simulink model "Ctrl_For_HRV_20260625"  (R2024b)
settings: Solver=ode4  StartTime=0.0  StopTime=22  FixedStep=0.02  RelTol=1e-3
InitFcn:
  | Parameter;
undefined symbols (not defined in the file or in its folder): CCI_DUI_AngleRate_Controller, CCI_DUI_FlowAngle_Controller, fhan, h_alpha, h_beta, h_miu, h_p, h_q, h_r, PNG_2026_6_23, r_alpha, r_beta, r_miu, r_p, r_q, r_r, xishu, xishu_D_0, xishu_L_0, xishu_l_0, xishu_m_0, xishu_n_0, xishu_Y_0
libraries: simulink x60
(part 3 of 8)

== system Ctrl_For_HRV_20260625/Vehicle_4/AngleRate_ESO_v4 ==
  Add{,1..5} (6 alike) : Sum  Inputs=+-
  Demux : Demux  Outputs=6
  Mux{,1..5} (6 alike) : Mux  Inputs=2
  Mux10 : Mux  Inputs=6
  S-Function : S-Function  FunctionName=fastloop_ESO  SFunctionDeploymentMode=off  EnableBusSupport=off
  Scope_p_hat : Scope
  Scope_p_hat_error : Scope
  Scope_phi_p_hat : Scope
  Scope_phi_p_hat_error : Scope
  Scope_phi_q_hat : Scope
  Scope_phi_q_hat_error : Scope
  Scope_phi_r_hat : Scope
  Scope_phi_r_hat_error : Scope
  Scope_q_hat : Scope
  Scope_q_hat_error : Scope
  Scope_r_hat : Scope
  Scope_r_hat_error : Scope
  tag scope: p_hat_v4=global, phi_p_hat_v4=global, phi_q_hat_v4=global, phi_r_hat_v4=global, q_hat_v4=global, r_hat_v4=global
  wires:
  Add5/1 -> Scope_phi_r_hat_error/1
  [phi_r_hat_v4] -> Add5/2
  [phi_r_v4] -> Add5/1
  Add4/1 -> Scope_phi_q_hat_error/1
  [phi_q_hat_v4] -> Add4/2
  [phi_q_v4] -> Add4/1
  Add3/1 -> Scope_phi_p_hat_error/1
  [phi_p_hat_v4] -> Add3/2
  [phi_p_v4] -> Add3/1
  Add2/1 -> Scope_r_hat_error/1
  [r_hat_v4] -> Add2/2
  [r_noise_v4] -> Add2/1
  Add1/1 -> Scope_q_hat_error/1
  [q_hat_v4] -> Add1/2
  [q_noise_v4] -> Add1/1
  Add/1 -> Scope_p_hat_error/1
  [p_hat_v4] -> Add/2
  [p_noise_v4] -> Add/1
  Mux3/1 -> Scope_phi_p_hat/1
  [phi_p_v4] -> Mux3/1
  [phi_p_hat_v4] -> Mux3/2
  [phi_q_v4] -> Mux4/1
  [phi_q_hat_v4] -> Mux4/2
  Mux4/1 -> Scope_phi_q_hat/1
  [phi_r_v4] -> Mux5/1
  [phi_r_hat_v4] -> Mux5/2
  Mux5/1 -> Scope_phi_r_hat/1
  Mux2/1 -> Scope_r_hat/1
  [r_hat_v4] -> Mux2/2
  [r_noise_v4] -> Mux2/1
  Mux1/1 -> Scope_q_hat/1
  [q_hat_v4] -> Mux1/2
  [q_noise_v4] -> Mux1/1
  [p_hat_v4] -> Mux/2
  [p_noise_v4] -> Mux/1
  Mux/1 -> Scope_p_hat/1
  [b_r_v4] -> Mux10/6
  [p_noise_v4] -> Mux10/1
  Demux/6 -> [phi_r_hat_v4]
  Mux10/1 -> S-Function/1
  Demux/4 -> [phi_p_hat_v4]
  Demux/3 -> [r_hat_v4]
  Demux/1 -> [p_hat_v4]
  Demux/5 -> [phi_q_hat_v4]
  S-Function/1 -> Demux/1
  [b_p_v4] -> Mux10/4
  Demux/2 -> [q_hat_v4]
  [q_noise_v4] -> Mux10/2
  [r_noise_v4] -> Mux10/3
  [b_q_v4] -> Mux10/5

== system Ctrl_For_HRV_20260625/Vehicle_4/Error_Model ==
  Delay : Delay  DelayLength=1
  Delay1 : Delay  DelayLength=1
  Delay2 : Delay  DelayLength=1
  Demux : Demux  Outputs=9
  Mux : Mux  Inputs=33
  S-Function : S-Function  FunctionName=Error_Model  SFunctionDeploymentMode=off  EnableBusSupport=off
  TD_alpha1 : Subsystem
  TD_alpha2 : Subsystem
  TD_alpha3 : Subsystem
  tag scope: dot_e_wd_1=global, dot_e_wd_2=global, dot_e_wd_3=global, e_alpha=global, e_beta=global, e_miu=global, e_w_1=global, e_w_2=global, e_w_3=global, e_wd_1=global, e_wd_2=global, e_wd_3=global
  wires:
  [theta] -> Mux/33
  [r] -> Mux/32
  [q] -> Mux/31
  [p] -> Mux/30
  [miu] -> Mux/29
  [beta] -> Mux/28
  [alpha] -> Mux/27
  [delta_r] -> Mux/3
  [delta_e] -> Mux/2
  [delta_a] -> Mux/1
  [dot_e_wd_3] -> Mux/26
  [dot_e_wd_2] -> Mux/25
  [dot_e_wd_1] -> Mux/24
  TD_alpha3/1(dot_e_wd_3) -> [dot_e_wd_3]
  [e_wd_3] -> TD_alpha3/1(e_wd_3)
  [e_wd_2] -> TD_alpha2/1(e_wd_2)
  TD_alpha2/1(dot_e_wd_2) -> [dot_e_wd_2]
  TD_alpha1/1(dot_e_wd_1) -> [dot_e_wd_1]
  [e_wd_1] -> TD_alpha1/1(e_wd_1)
  Delay2/1 -> Mux/23
  [e_wd_3] -> Delay2/1
  [e_wd_2] -> Delay1/1
  Delay1/1 -> Mux/22
  Delay/1 -> Mux/21
  [e_wd_1] -> Delay/1
  Demux/7 -> [e_wd_1]
  Demux/8 -> [e_wd_2]
  Demux/9 -> [e_wd_3]
  Demux/6 -> [e_w_3]
  Demux/5 -> [e_w_2]
  Demux/4 -> [e_w_1]
  Demux/3 -> [e_miu]
  Demux/2 -> [e_beta]
  Demux/1 -> [e_alpha]
  S-Function/1 -> Demux/1
  [ddot_miu_c] -> Mux/20
  [ddot_beta_c] -> Mux/19
  [ddot_alpha_c] -> Mux/18
  [dot_alpha_c] -> Mux/15
  [dot_beta_c] -> Mux/16
  [dot_miu_c] -> Mux/17
  [miu_c] -> Mux/14
  [beta_c] -> Mux/13
  [alpha_c] -> Mux/12
  [V] -> Mux/11
  [H] -> Mux/10
  [C_m_d] -> Mux/8
  [C_n_d] -> Mux/9
  [C_Y_d] -> Mux/6
  [C_L_d] -> Mux/4
  [C_D_d] -> Mux/5
  [C_l_d] -> Mux/7
  Mux/1 -> S-Function/1

== system Ctrl_For_HRV_20260625/Vehicle_4/FlowAngle_Controller_v4 ==
  alpha_d : Inport
  beta_d : Inport  Port=2
  miu_d : Inport  Port=3
  Demux : Demux  Outputs=9
  From12 : From  Commented=on  GotoTag=dot_alpha_c  TagVisibility=global
  From13 : From  Commented=on  GotoTag=dot_beta_c  TagVisibility=global
  From14 : From  Commented=on  GotoTag=dot_miu_c  TagVisibility=global
  Goto6 : Goto  Commented=on  GotoTag=ddot_alpha_c  TagVisibility=global
  Goto7 : Goto  Commented=on  GotoTag=ddot_beta_c  TagVisibility=global
  Goto8 : Goto  Commented=on  GotoTag=ddot_miu_c  TagVisibility=global
  Interpreted MATLAB Function : MATLABFcn  MATLABFcn=CCI_DUI_FlowAngle_Controller(u(1),u(2),u(3),u(4),u(5),u(6),u(7),u(8),u(9),u(10),u(11),u(12),u(13),u(14),u(15),u(16),u(17),u(18))  OutputDimensions=9
  Mux : Mux  Inputs=18
  Mux1 : Mux  Inputs=3
  Mux2 : Mux  Inputs=3
  Scope_CCI_FlowAngle : Scope
  Scope_DUI_FlowAngle : Scope
  Scope_alpha_d : Scope
  Scope_beta_d : Scope
  Scope_miu_d : Scope
  TD_alpha : Subsystem
  TD_alpha2 : Subsystem
  TD_alpha3 : Subsystem  Commented=on
  TD_alpha4 : Subsystem  Commented=on
  TD_beta : Subsystem
  TD_beta1 : Subsystem
  TD_beta2 : Subsystem
  TD_dotalpha1 : Subsystem  Commented=on
  TD_miu : Subsystem
  p_d : Outport
  q_d : Outport  Port=2
  r_d : Outport  Port=3
  tag scope: alpha_c_v4=global, beta_c_v4=global, dot_alpha_c_v4=global, dot_beta_c_v4=global, dot_miu_c_v4=global, miu_c_v4=global
  wires:
  Demux/7 -> Mux2/1
  Demux/9 -> Mux2/3
  Demux/8 -> Mux2/2
  Mux2/1 -> Scope_DUI_FlowAngle/1
  Mux1/1 -> Scope_CCI_FlowAngle/1
  Demux/6 -> Mux1/3
  Demux/5 -> Mux1/2
  Demux/4 -> Mux1/1
  TD_alpha/1(alpha_c) -> Mux/13, [alpha_c_v4]
  TD_alpha4/1(ddot_miu_c) -> Goto8/1
  From14/1 -> TD_alpha4/1(dot_miu_c)
  TD_alpha3/1(ddot_beta_c) -> Goto7/1
  From13/1 -> TD_alpha3/1(dot_beta_c)
  TD_dotalpha1/1(ddot_alpha_c) -> Goto6/1
  From12/1 -> TD_dotalpha1/1(dot_alpha_c)
  [phi_miu_hat_v4] -> Mux/12
  [phi_beta_hat_v4] -> Mux/11
  [phi_alpha_hat_v4] -> Mux/10
  TD_miu/2(miu_c_dot) -> Mux/18, [dot_miu_c_v4]
  TD_miu/1(miu_c) -> Mux/17, [miu_c_v4]
  miu_d/1 -> TD_miu/1(miu_d), Scope_miu_d/1
  TD_beta/2(beta_c_dot) -> Mux/16, [dot_beta_c_v4]
  TD_beta/1(beta_c) -> Mux/15, [beta_c_v4]
  beta_d/1 -> TD_beta/1(beta_d), Scope_beta_d/1
  TD_alpha/2(alpha_c_dot) -> [dot_alpha_c_v4], Mux/14
  alpha_d/1 -> TD_alpha/1(alpha_d), Scope_alpha_d/1
  Demux/3 -> r_d/1
  Demux/2 -> q_d/1
  Demux/1 -> p_d/1
  Interpreted MATLAB Function/1 -> Demux/1
  Mux/1 -> Interpreted MATLAB Function/1
  [theta_v4] -> Mux/9
  [delta_a_v4] -> Mux/6
  [delta_e_v4] -> Mux/7
  [delta_r_v4] -> Mux/8
  [miu_noise_v4] -> Mux/5
  [beta_noise_v4] -> Mux/4
  [alpha_noise_v4] -> Mux/3
  [V_v4] -> Mux/2
  [H_v4] -> Mux/1

== system Ctrl_For_HRV_20260625/Vehicle_4/FlowAngle_ESO_v4 ==
  Add{,1..5} (6 alike) : Sum  Inputs=+-
  Demux : Demux  Outputs=6
  Mux{,1..5} (6 alike) : Mux  Inputs=2
  Mux10 : Mux  Inputs=6
  S-Function : S-Function  FunctionName=slowloop_ESO  SFunctionDeploymentMode=off  EnableBusSupport=off
  Scope_alpha_hat : Scope
  Scope_alpha_hat_error : Scope
  Scope_beta_hat : Scope
  Scope_beta_hat_error : Scope
  Scope_miu_hat : Scope
  Scope_miu_hat_error : Scope
  Scope_phi_alpha_hat : Scope
  Scope_phi_alpha_hat_error : Scope
  Scope_phi_beta_hat : Scope
  Scope_phi_beta_hat_error : Scope
  Scope_phi_miu_hat : Scope
  Scope_phi_miu_hat_error : Scope
  tag scope: alpha_hat_v4=global, beta_hat_v4=global, miu_hat_v4=global, phi_alpha_hat_v4=global, phi_beta_hat_v4=global, phi_miu_hat_v4=global
  wires:
  [phi_miu_hat_v4] -> Add5/2
  [phi_miu_v4] -> Add5/1
  Add5/1 -> Scope_phi_miu_hat_error/1
  Add4/1 -> Scope_phi_beta_hat_error/1
  [phi_beta_hat_v4] -> Add4/2
  [phi_beta_v4] -> Add4/1
  Add3/1 -> Scope_phi_alpha_hat_error/1
  [phi_alpha_hat_v4] -> Add3/2
  [phi_alpha_v4] -> Add3/1
  Add2/1 -> Scope_miu_hat_error/1
  [miu_hat_v4] -> Add2/2
  [miu_noise_v4] -> Add2/1
  Add1/1 -> Scope_beta_hat_error/1
  [beta_hat_v4] -> Add1/2
  [beta_noise_v4] -> Add1/1
  Add/1 -> Scope_alpha_hat_error/1
  [alpha_hat_v4] -> Add/2
  [alpha_noise_v4] -> Add/1
  Mux3/1 -> Scope_phi_alpha_hat/1
  [phi_alpha_v4] -> Mux3/1
  [phi_alpha_hat_v4] -> Mux3/2
  [phi_beta_v4] -> Mux4/1
  [phi_beta_hat_v4] -> Mux4/2
  Mux4/1 -> Scope_phi_beta_hat/1
  [phi_miu_v4] -> Mux5/1
  [phi_miu_hat_v4] -> Mux5/2
  Mux5/1 -> Scope_phi_miu_hat/1
  Mux2/1 -> Scope_miu_hat/1
  [miu_hat_v4] -> Mux2/2
  [miu_noise_v4] -> Mux2/1
  Mux1/1 -> Scope_beta_hat/1
  [beta_hat_v4] -> Mux1/2
  [beta_noise_v4] -> Mux1/1
  [alpha_hat_v4] -> Mux/2
  [alpha_noise_v4] -> Mux/1
  Mux/1 -> Scope_alpha_hat/1
  [b_miu_v4] -> Mux10/6
  [alpha_noise_v4] -> Mux10/1
  Demux/6 -> [phi_miu_hat_v4]
  Mux10/1 -> S-Function/1
  Demux/4 -> [phi_alpha_hat_v4]
  Demux/3 -> [miu_hat_v4]
  Demux/1 -> [alpha_hat_v4]
  Demux/5 -> [phi_beta_hat_v4]
  S-Function/1 -> Demux/1
  [b_alpha_v4] -> Mux10/4
  Demux/2 -> [beta_hat_v4]
  [beta_noise_v4] -> Mux10/2
  [miu_noise_v4] -> Mux10/3
  [b_beta_v4] -> Mux10/5

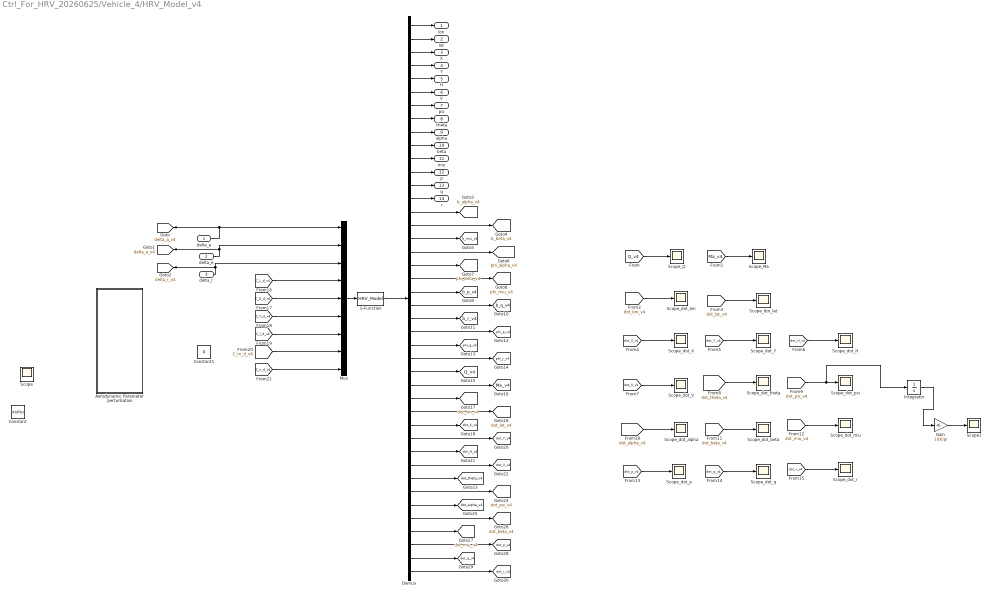
== system Ctrl_For_HRV_20260625/Vehicle_4/HRV_Model_v4 ==
  delta_a : Inport
  delta_e : Inport  Port=2
  delta_r : Inport  Port=3
  Aerodynamic Parameter perturbation : Subsystem
  Constant : Constant  Value=xishu  SampleTime=-1
  Constant1 : Constant  Value=0
  Demux : Demux  Outputs=14 + 12 + 2 + 14
  Gain : Gain  Gain=180/pi
  Integrator : Integrator  InitialCondition=[0 0 450 350 0 0 0.0349065850398866 0 0 0 0 0 0 0 0 0 0 0 0 0 0 0 0 0 0 0 0 0 0 0 0 0 0 0 0 0 0 0 0 0 0 0]
  Mux : Mux  Inputs=9
  S-Function : S-Function  FunctionName=HRV_Model  SFunctionDeploymentMode=off  EnableBusSupport=off
  Scope : Scope
  Scope1 : Scope
  Scope_Ma : Scope
  Scope_Q : Scope
  Scope_dot_H : Scope
  Scope_dot_V : Scope
  Scope_dot_X : Scope
  Scope_dot_Y : Scope
  Scope_dot_alpha : Scope
  Scope_dot_beta : Scope
  Scope_dot_lat : Scope
  Scope_dot_lon : Scope
  Scope_dot_miu : Scope
  Scope_dot_p : Scope
  Scope_dot_psi : Scope
  Scope_dot_q : Scope
  Scope_dot_r : Scope
  Scope_dot_theta : Scope
  lon : Outport
  lat : Outport  Port=2
  X : Outport  Port=3
  Y : Outport  Port=4
  H : Outport  Port=5
  V : Outport  Port=6
  psi : Outport  Port=7
  theta : Outport  Port=8
  alpha : Outport  Port=9
  beta : Outport  Port=10
  miu : Outport  Port=11
  p : Outport  Port=12
  q : Outport  Port=13
  r : Outport  Port=14
  tag scope: Ma_v4=global, Q_v4=global, b_alpha_v4=global, b_beta_v4=global, b_miu_v4=global, b_p_v4=global, b_q_v4=global, b_r_v4=global, delta_a_v4=global, delta_e_v4=global, delta_r_v4=global, dot_H_v4=global, dot_V_v4=global, dot_X_v4=global, dot_Y_v4=global, dot_alpha_v4=global, dot_beta_v4=global, dot_lat_v4=global, dot_lon_v4=global, dot_miu_v4=global, dot_p_v4=global, dot_psi_v4=global, dot_q_v4=global, dot_r_v4=global, dot_theta_v4=global, phi_alpha_v4=global, phi_beta_v4=global, phi_miu_v4=global, phi_p_v4=global, phi_q_v4=global, phi_r_v4=global
  wires:
  Gain/1 -> Scope1/1
  Integrator/1 -> Gain/1
  [C_n_d_v4] -> Mux/9
  [C_m_d_v4] -> Mux/8
  [C_l_d_v4] -> Mux/7
  [C_Y_d_v4] -> Mux/6
  [C_D_d_v4] -> Mux/5
  [C_L_d_v4] -> Mux/4
  [dot_p_v4] -> Scope_dot_p/1
  [dot_q_v4] -> Scope_dot_q/1
  [dot_r_v4] -> Scope_dot_r/1
  [dot_miu_v4] -> Scope_dot_miu/1
  [dot_beta_v4] -> Scope_dot_beta/1
  [dot_alpha_v4] -> Scope_dot_alpha/1
  [dot_psi_v4] -> Scope_dot_psi/1, Integrator/1
  [dot_theta_v4] -> Scope_dot_theta/1
  [dot_V_v4] -> Scope_dot_V/1
  [dot_H_v4] -> Scope_dot_H/1
  [dot_Y_v4] -> Scope_dot_Y/1
  [dot_X_v4] -> Scope_dot_X/1
  [dot_lat_v4] -> Scope_dot_lat/1
  [dot_lon_v4] -> Scope_dot_lon/1
  [Ma_v4] -> Scope_Ma/1
  [Q_v4] -> Scope_Q/1
  Demux/42 -> [dot_r_v4]
  Demux/41 -> [dot_q_v4]
  Demux/40 -> [dot_p_v4]
  Demux/38 -> [dot_beta_v4]
  Demux/39 -> [dot_miu_v4]
  Demux/33 -> [dot_H_v4]
  Demux/35 -> [dot_theta_v4]
  Demux/34 -> [dot_V_v4]
  Demux/36 -> [dot_psi_v4]
  Demux/37 -> [dot_alpha_v4]
  Demux/32 -> [dot_Y_v4]
  Demux/31 -> [dot_X_v4]
  Demux/29 -> [dot_lon_v4]
  Demux/30 -> [dot_lat_v4]
  Demux/28 -> [Ma_v4]
  Demux/27 -> [Q_v4]
  Demux/26 -> [phi_r_v4]
  Demux/25 -> [phi_q_v4]
  Demux/24 -> [phi_p_v4]
  Demux/23 -> [b_r_v4]
  Demux/19 -> [phi_beta_v4]
  Demux/20 -> [phi_miu_v4]
  Demux/22 -> [b_q_v4]
  Demux/21 -> [b_p_v4]
  Demux/17 -> [b_miu_v4]
  Demux/18 -> [phi_alpha_v4]
  Demux/16 -> [b_beta_v4]
  Demux/15 -> [b_alpha_v4]
  Demux/4 -> Y/1
  delta_a/1 -> Mux/1, [delta_a_v4]
  Demux/13 -> q/1
  delta_r/1 -> Mux/3, [delta_r_v4]
  Demux/14 -> r/1
  Demux/6 -> V/1
  delta_e/1 -> Mux/2, [delta_e_v4]
  Demux/5 -> H/1
  Demux/12 -> p/1
  Demux/9 -> alpha/1
  Demux/10 -> beta/1
  Demux/11 -> miu/1
  Demux/7 -> psi/1
  Demux/3 -> X/1
  Demux/2 -> lat/1
  Demux/1 -> lon/1
  S-Function/1 -> Demux/1
  Mux/1 -> S-Function/1
  Demux/8 -> theta/1

== system Ctrl_For_HRV_20260625/Vehicle_4/PNG ==
  Delay : Delay  DelayLength=1
  Demux : Demux  Outputs=3
  MATLAB Function : MATLAB Function  TreatAsAtomicUnit=on
  MATLAB Function1 : MATLAB Function  TreatAsAtomicUnit=on  SystemSampleTime=0.02
  MATLAB Function2 : MATLAB Function  TreatAsAtomicUnit=on
  Mux : Mux  Inputs=7+2
  PNG : MATLABFcn  MATLABFcn=PNG_2026_6_23(u)  OutputDimensions=3
  Scope{,1..4} (5 alike) : Scope
  Scope5 : Scope  NumInputPorts=2
  tag scope: alpha_cmd=global, f_psi=global, miu_cmd=global
  wires:
  Delay/1 -> MATLAB Function1/6(miu_last)
  [theta] -> Mux/9
  [f_psi] -> Mux/8
  MATLAB Function2/1(f_psi) -> [f_psi]
  [H] -> MATLAB Function2/5(H)
  [lat] -> MATLAB Function2/4(lat)
  [psi] -> MATLAB Function2/3(psi)
  [theta] -> MATLAB Function2/2(theta)
  [V] -> MATLAB Function2/1(V)
  Demux/3 -> Scope5/1
  [Q] -> Mux/7
  MATLAB Function1/2(miu_cmd) -> [miu_cmd], Scope3/1, Delay/1
  MATLAB Function1/1(alpha_cmd) -> [alpha_cmd], Scope2/1
  [Ma] -> MATLAB Function1/5(Ma)
  [H] -> MATLAB Function1/4(H)
  [Q] -> MATLAB Function1/3(Q)
  [nz_cmd] -> MATLAB Function1/2(nz_cmd)
  [ny_cmd] -> MATLAB Function1/1(ny_cmd)
  [nz_cmd] -> Scope1/1
  [ny_cmd] -> Scope/1
  Demux/2 -> [nz_cmd], Scope5/2
  Demux/1 -> [ny_cmd]
  PNG/1 -> Demux/1
  [V_target] -> Mux/6
  [Position_target] -> Mux/5
  MATLAB Function/1(v) -> Mux/4, Scope4/1
  [psi] -> MATLAB Function/3(psi)
  [theta] -> MATLAB Function/2(theta)
  [V] -> MATLAB Function/1(V)
  [H] -> Mux/3
  [Y] -> Mux/2
  [X] -> Mux/1
  Mux/1 -> PNG/1

== system Ctrl_For_HRV_20260625/Vehicle_4/actuator1_v4 ==
  delta_e_d : Inport
  Gain : Gain  Gain=50
  Integrator : Integrator
  Saturation : Saturate  UpperLimit=90  LowerLimit=-90
  Saturation1 : Saturate  UpperLimit=30  LowerLimit=-30
  Sum : Sum  Inputs=|+-
  delta_e : Outport
  wires:
  Saturation/1 -> Integrator/1
  Sum/1 -> Gain/1
  Integrator/1 -> Saturation1/1, Sum/2
  delta_e_d/1 -> Sum/1
  Gain/1 -> Saturation/1
  Saturation1/1 -> delta_e/1

== system Ctrl_For_HRV_20260625/Vehicle_4/actuator2_v4 ==
  delta_r_d : Inport
  Gain : Gain  Gain=50
  Integrator : Integrator
  Saturation : Saturate  UpperLimit=90  LowerLimit=-90
  Saturation1 : Saturate  UpperLimit=30  LowerLimit=-30
  Sum : Sum  Inputs=|+-
  delta_r : Outport
  wires:
  Saturation1/1 -> delta_r/1
  Gain/1 -> Saturation/1
  delta_r_d/1 -> Sum/1
  Integrator/1 -> Sum/2, Saturation1/1
  Sum/1 -> Gain/1
  Saturation/1 -> Integrator/1

== system Ctrl_For_HRV_20260625/Vehicle_4/actuator_v4 ==
  delta_a_d : Inport
  Gain : Gain  Gain=50
  Integrator : Integrator
  Saturation : Saturate  UpperLimit=90  LowerLimit=-90
  Saturation1 : Saturate  UpperLimit=30  LowerLimit=-30
  Sum : Sum  Inputs=|+-
  delta_a : Outport
  wires:
  Saturation1/1 -> delta_a/1
  Gain/1 -> Saturation/1
  delta_a_d/1 -> Sum/1
  Integrator/1 -> Sum/2, Saturation1/1
  Sum/1 -> Gain/1
  Saturation/1 -> Integrator/1

== system Ctrl_For_HRV_20260625/Vehicle_5/AngleRate_Controller_v5 ==
  p_d : Inport
  q_d : Inport  Port=2
  r_d : Inport  Port=3
  Demux : Demux  Outputs=9
  Interpreted MATLAB Function : MATLABFcn  MATLABFcn=CCI_DUI_AngleRate_Controller(u(1),u(2),u(3),u(4),u(5),u(6),u(7),u(8),u(9),u(10),u(11),u(12),u(13),u(14),u(15),u(16),u(17),u(18),u(19),u(20),u(21),u(22),u(23))  OutputDimensions=9
  Mux : Mux  Inputs=23
  Mux1 : Mux  Inputs=3
  Mux2 : Mux  Inputs=3
  Scope2 : Scope
  Scope_CCI_AngleRate : Scope
  Scope_DUI_AngleRate : Scope
  Scope_p_d : Scope
  Scope_q_d : Scope
  Scope_r_d : Scope
  TD_p : Subsystem
  TD_q : Subsystem
  TD_r : Subsystem
  delta_a_d : Outport
  delta_e_d : Outport  Port=2
  delta_r_d : Outport  Port=3
  tag scope: delta_a_d_v5=global, delta_e_d_v5=global, delta_r_d_v5=global, p_c_v5=global, q_c_v5=global, r_c_v5=global
  wires:
  Mux2/1 -> Scope_DUI_AngleRate/1
  Demux/9 -> Mux2/3
  Demux/8 -> Mux2/2
  Demux/7 -> Mux2/1
  Mux1/1 -> Scope_CCI_AngleRate/1
  Demux/6 -> Mux1/3
  Demux/5 -> Mux1/2
  Demux/4 -> Mux1/1
  [miu_c_v5] -> Mux/23
  [beta_c_v5] -> Mux/22
  [alpha_c_v5] -> Mux/21
  [phi_r_hat_v5] -> Mux/14
  [phi_q_hat_v5] -> Mux/13
  [phi_p_hat_v5] -> Mux/12
  p_d/1 -> TD_p/1(p_d), Scope_p_d/1
  q_d/1 -> TD_q/1(q_d), Scope_q_d/1
  Demux/1 -> delta_a_d/1, [delta_a_d_v5]
  Demux/2 -> delta_e_d/1, [delta_e_d_v5]
  r_d/1 -> TD_r/1(r_d), Scope_r_d/1
  Demux/3 -> [delta_r_d_v5], delta_r_d/1
  TD_p/1(p_c) -> Mux/15, [p_c_v5]
  [delta_e_v5] -> Mux/7
  [delta_r_v5] -> Mux/8
  [delta_a_v5] -> Mux/6
  Interpreted MATLAB Function/1 -> Demux/1
  Mux/1 -> Interpreted MATLAB Function/1
  [alpha_noise_v5] -> Mux/3
  [V_v5] -> Mux/2
  [p_noise_v5] -> Mux/9
  [H_v5] -> Mux/1
  [r_noise_v5] -> Mux/11
  TD_r/2(r_c_dot) -> Mux/20
  TD_q/1(q_c) -> Mux/17, [q_c_v5]
  [q_noise_v5] -> Mux/10
  TD_q/2(q_c_dot) -> Mux/18
  TD_p/2(p_c_dot) -> Mux/16
  TD_r/1(r_c) -> Mux/19, [r_c_v5]
  [beta_noise_v5] -> Mux/4
  [miu_noise_v5] -> Mux/5

== system Ctrl_For_HRV_20260625/Vehicle_5/AngleRate_ESO_v5 ==
  Add{,1..5} (6 alike) : Sum  Inputs=+-
  Demux : Demux  Outputs=6
  Mux{,1..5} (6 alike) : Mux  Inputs=2
  Mux10 : Mux  Inputs=6
  S-Function : S-Function  FunctionName=fastloop_ESO  SFunctionDeploymentMode=off  EnableBusSupport=off
  Scope_p_hat : Scope
  Scope_p_hat_error : Scope
  Scope_phi_p_hat : Scope
  Scope_phi_p_hat_error : Scope
  Scope_phi_q_hat : Scope
  Scope_phi_q_hat_error : Scope
  Scope_phi_r_hat : Scope
  Scope_phi_r_hat_error : Scope
  Scope_q_hat : Scope
  Scope_q_hat_error : Scope
  Scope_r_hat : Scope
  Scope_r_hat_error : Scope
  tag scope: p_hat_v5=global, phi_p_hat_v5=global, phi_q_hat_v5=global, phi_r_hat_v5=global, q_hat_v5=global, r_hat_v5=global
  wires:
  Add5/1 -> Scope_phi_r_hat_error/1
  [phi_r_hat_v5] -> Add5/2
  [phi_r_v5] -> Add5/1
  Add4/1 -> Scope_phi_q_hat_error/1
  [phi_q_hat_v5] -> Add4/2
  [phi_q_v5] -> Add4/1
  Add3/1 -> Scope_phi_p_hat_error/1
  [phi_p_hat_v5] -> Add3/2
  [phi_p_v5] -> Add3/1
  Add2/1 -> Scope_r_hat_error/1
  [r_hat_v5] -> Add2/2
  [r_noise_v5] -> Add2/1
  Add1/1 -> Scope_q_hat_error/1
  [q_hat_v5] -> Add1/2
  [q_noise_v5] -> Add1/1
  Add/1 -> Scope_p_hat_error/1
  [p_hat_v5] -> Add/2
  [p_noise_v5] -> Add/1
  Mux3/1 -> Scope_phi_p_hat/1
  [phi_p_v5] -> Mux3/1
  [phi_p_hat_v5] -> Mux3/2
  [phi_q_v5] -> Mux4/1
  [phi_q_hat_v5] -> Mux4/2
  Mux4/1 -> Scope_phi_q_hat/1
  [phi_r_v5] -> Mux5/1
  [phi_r_hat_v5] -> Mux5/2
  Mux5/1 -> Scope_phi_r_hat/1
  Mux2/1 -> Scope_r_hat/1
  [r_hat_v5] -> Mux2/2
  [r_noise_v5] -> Mux2/1
  Mux1/1 -> Scope_q_hat/1
  [q_hat_v5] -> Mux1/2
  [q_noise_v5] -> Mux1/1
  [p_hat_v5] -> Mux/2
  [p_noise_v5] -> Mux/1
  Mux/1 -> Scope_p_hat/1
  [b_r_v5] -> Mux10/6
  [p_noise_v5] -> Mux10/1
  Demux/6 -> [phi_r_hat_v5]
  Mux10/1 -> S-Function/1
  Demux/4 -> [phi_p_hat_v5]
  Demux/3 -> [r_hat_v5]
  Demux/1 -> [p_hat_v5]
  Demux/5 -> [phi_q_hat_v5]
  S-Function/1 -> Demux/1
  [b_p_v5] -> Mux10/4
  Demux/2 -> [q_hat_v5]
  [q_noise_v5] -> Mux10/2
  [r_noise_v5] -> Mux10/3
  [b_q_v5] -> Mux10/5

== system Ctrl_For_HRV_20260625/Vehicle_5/Error_Model ==
  Delay : Delay  DelayLength=1
  Delay1 : Delay  DelayLength=1
  Delay2 : Delay  DelayLength=1
  Demux : Demux  Outputs=9
  Mux : Mux  Inputs=33
  S-Function : S-Function  FunctionName=Error_Model  SFunctionDeploymentMode=off  EnableBusSupport=off
  TD_alpha1 : Subsystem
  TD_alpha2 : Subsystem
  TD_alpha3 : Subsystem
  tag scope: dot_e_wd_1=global, dot_e_wd_2=global, dot_e_wd_3=global, e_alpha=global, e_beta=global, e_miu=global, e_w_1=global, e_w_2=global, e_w_3=global, e_wd_1=global, e_wd_2=global, e_wd_3=global
  wires:
  [theta] -> Mux/33
  [r] -> Mux/32
  [q] -> Mux/31
  [p] -> Mux/30
  [miu] -> Mux/29
  [beta] -> Mux/28
  [alpha] -> Mux/27
  [delta_r] -> Mux/3
  [delta_e] -> Mux/2
  [delta_a] -> Mux/1
  [dot_e_wd_3] -> Mux/26
  [dot_e_wd_2] -> Mux/25
  [dot_e_wd_1] -> Mux/24
  TD_alpha3/1(dot_e_wd_3) -> [dot_e_wd_3]
  [e_wd_3] -> TD_alpha3/1(e_wd_3)
  [e_wd_2] -> TD_alpha2/1(e_wd_2)
  TD_alpha2/1(dot_e_wd_2) -> [dot_e_wd_2]
  TD_alpha1/1(dot_e_wd_1) -> [dot_e_wd_1]
  [e_wd_1] -> TD_alpha1/1(e_wd_1)
  Delay2/1 -> Mux/23
  [e_wd_3] -> Delay2/1
  [e_wd_2] -> Delay1/1
  Delay1/1 -> Mux/22
  Delay/1 -> Mux/21
  [e_wd_1] -> Delay/1
  Demux/7 -> [e_wd_1]
  Demux/8 -> [e_wd_2]
  Demux/9 -> [e_wd_3]
  Demux/6 -> [e_w_3]
  Demux/5 -> [e_w_2]
  Demux/4 -> [e_w_1]
  Demux/3 -> [e_miu]
  Demux/2 -> [e_beta]
  Demux/1 -> [e_alpha]
  S-Function/1 -> Demux/1
  [ddot_miu_c] -> Mux/20
  [ddot_beta_c] -> Mux/19
  [ddot_alpha_c] -> Mux/18
  [dot_alpha_c] -> Mux/15
  [dot_beta_c] -> Mux/16
  [dot_miu_c] -> Mux/17
  [miu_c] -> Mux/14
  [beta_c] -> Mux/13
  [alpha_c] -> Mux/12
  [V] -> Mux/11
  [H] -> Mux/10
  [C_m_d] -> Mux/8
  [C_n_d] -> Mux/9
  [C_Y_d] -> Mux/6
  [C_L_d] -> Mux/4
  [C_D_d] -> Mux/5
  [C_l_d] -> Mux/7
  Mux/1 -> S-Function/1

== system Ctrl_For_HRV_20260625/Vehicle_5/FlowAngle_Controller_v5 ==
  alpha_d : Inport
  beta_d : Inport  Port=2
  miu_d : Inport  Port=3
  Demux : Demux  Outputs=9
  From12 : From  Commented=on  GotoTag=dot_alpha_c  TagVisibility=global
  From13 : From  Commented=on  GotoTag=dot_beta_c  TagVisibility=global
  From14 : From  Commented=on  GotoTag=dot_miu_c  TagVisibility=global
  Goto6 : Goto  Commented=on  GotoTag=ddot_alpha_c  TagVisibility=global
  Goto7 : Goto  Commented=on  GotoTag=ddot_beta_c  TagVisibility=global
  Goto8 : Goto  Commented=on  GotoTag=ddot_miu_c  TagVisibility=global
  Interpreted MATLAB Function : MATLABFcn  MATLABFcn=CCI_DUI_FlowAngle_Controller(u(1),u(2),u(3),u(4),u(5),u(6),u(7),u(8),u(9),u(10),u(11),u(12),u(13),u(14),u(15),u(16),u(17),u(18))  OutputDimensions=9
  Mux : Mux  Inputs=18
  Mux1 : Mux  Inputs=3
  Mux2 : Mux  Inputs=3
  Scope_CCI_FlowAngle : Scope
  Scope_DUI_FlowAngle : Scope
  Scope_alpha_d : Scope
  Scope_beta_d : Scope
  Scope_miu_d : Scope
  TD_alpha : Subsystem
  TD_alpha2 : Subsystem
  TD_alpha3 : Subsystem  Commented=on
  TD_alpha4 : Subsystem  Commented=on
  TD_beta : Subsystem
  TD_beta1 : Subsystem
  TD_beta2 : Subsystem
  TD_dotalpha1 : Subsystem  Commented=on
  TD_miu : Subsystem
  p_d : Outport
  q_d : Outport  Port=2
  r_d : Outport  Port=3
  tag scope: alpha_c_v5=global, beta_c_v5=global, dot_alpha_c_v5=global, dot_beta_c_v5=global, dot_miu_c_v5=global, miu_c_v5=global
  wires:
  Demux/7 -> Mux2/1
  Demux/9 -> Mux2/3
  Demux/8 -> Mux2/2
  Mux2/1 -> Scope_DUI_FlowAngle/1
  Mux1/1 -> Scope_CCI_FlowAngle/1
  Demux/6 -> Mux1/3
  Demux/5 -> Mux1/2
  Demux/4 -> Mux1/1
  TD_alpha/1(alpha_c) -> Mux/13, [alpha_c_v5]
  TD_alpha4/1(ddot_miu_c) -> Goto8/1
  From14/1 -> TD_alpha4/1(dot_miu_c)
  TD_alpha3/1(ddot_beta_c) -> Goto7/1
  From13/1 -> TD_alpha3/1(dot_beta_c)
  TD_dotalpha1/1(ddot_alpha_c) -> Goto6/1
  From12/1 -> TD_dotalpha1/1(dot_alpha_c)
  [phi_miu_hat_v5] -> Mux/12
  [phi_beta_hat_v5] -> Mux/11
  [phi_alpha_hat_v5] -> Mux/10
  TD_miu/2(miu_c_dot) -> Mux/18, [dot_miu_c_v5]
  TD_miu/1(miu_c) -> Mux/17, [miu_c_v5]
  miu_d/1 -> TD_miu/1(miu_d), Scope_miu_d/1
  TD_beta/2(beta_c_dot) -> Mux/16, [dot_beta_c_v5]
  TD_beta/1(beta_c) -> Mux/15, [beta_c_v5]
  beta_d/1 -> TD_beta/1(beta_d), Scope_beta_d/1
  TD_alpha/2(alpha_c_dot) -> [dot_alpha_c_v5], Mux/14
  alpha_d/1 -> TD_alpha/1(alpha_d), Scope_alpha_d/1
  Demux/3 -> r_d/1
  Demux/2 -> q_d/1
  Demux/1 -> p_d/1
  Interpreted MATLAB Function/1 -> Demux/1
  Mux/1 -> Interpreted MATLAB Function/1
  [theta_v5] -> Mux/9
  [delta_a_v5] -> Mux/6
  [delta_e_v5] -> Mux/7
  [delta_r_v5] -> Mux/8
  [miu_noise_v5] -> Mux/5
  [beta_noise_v5] -> Mux/4
  [alpha_noise_v5] -> Mux/3
  [V_v5] -> Mux/2
  [H_v5] -> Mux/1

== system Ctrl_For_HRV_20260625/Vehicle_5/FlowAngle_ESO_v5 ==
  Add{,1..5} (6 alike) : Sum  Inputs=+-
  Demux : Demux  Outputs=6
  Mux{,1..5} (6 alike) : Mux  Inputs=2
  Mux10 : Mux  Inputs=6
  S-Function : S-Function  FunctionName=slowloop_ESO  SFunctionDeploymentMode=off  EnableBusSupport=off
  Scope_alpha_hat : Scope
  Scope_alpha_hat_error : Scope
  Scope_beta_hat : Scope
  Scope_beta_hat_error : Scope
  Scope_miu_hat : Scope
  Scope_miu_hat_error : Scope
  Scope_phi_alpha_hat : Scope
  Scope_phi_alpha_hat_error : Scope
  Scope_phi_beta_hat : Scope
  Scope_phi_beta_hat_error : Scope
  Scope_phi_miu_hat : Scope
  Scope_phi_miu_hat_error : Scope
  tag scope: alpha_hat_v5=global, beta_hat_v5=global, miu_hat_v5=global, phi_alpha_hat_v5=global, phi_beta_hat_v5=global, phi_miu_hat_v5=global
  wires:
  [phi_miu_hat_v5] -> Add5/2
  [phi_miu_v5] -> Add5/1
  Add5/1 -> Scope_phi_miu_hat_error/1
  Add4/1 -> Scope_phi_beta_hat_error/1
  [phi_beta_hat_v5] -> Add4/2
  [phi_beta_v5] -> Add4/1
  Add3/1 -> Scope_phi_alpha_hat_error/1
  [phi_alpha_hat_v5] -> Add3/2
  [phi_alpha_v5] -> Add3/1
  Add2/1 -> Scope_miu_hat_error/1
  [miu_hat_v5] -> Add2/2
  [miu_noise_v5] -> Add2/1
  Add1/1 -> Scope_beta_hat_error/1
  [beta_hat_v5] -> Add1/2
  [beta_noise_v5] -> Add1/1
  Add/1 -> Scope_alpha_hat_error/1
  [alpha_hat_v5] -> Add/2
  [alpha_noise_v5] -> Add/1
  Mux3/1 -> Scope_phi_alpha_hat/1
  [phi_alpha_v5] -> Mux3/1
  [phi_alpha_hat_v5] -> Mux3/2
  [phi_beta_v5] -> Mux4/1
  [phi_beta_hat_v5] -> Mux4/2
  Mux4/1 -> Scope_phi_beta_hat/1
  [phi_miu_v5] -> Mux5/1
  [phi_miu_hat_v5] -> Mux5/2
  Mux5/1 -> Scope_phi_miu_hat/1
  Mux2/1 -> Scope_miu_hat/1
  [miu_hat_v5] -> Mux2/2
  [miu_noise_v5] -> Mux2/1
  Mux1/1 -> Scope_beta_hat/1
  [beta_hat_v5] -> Mux1/2
  [beta_noise_v5] -> Mux1/1
  [alpha_hat_v5] -> Mux/2
  [alpha_noise_v5] -> Mux/1
  Mux/1 -> Scope_alpha_hat/1
  [b_miu_v5] -> Mux10/6
  [alpha_noise_v5] -> Mux10/1
  Demux/6 -> [phi_miu_hat_v5]
  Mux10/1 -> S-Function/1
  Demux/4 -> [phi_alpha_hat_v5]
  Demux/3 -> [miu_hat_v5]
  Demux/1 -> [alpha_hat_v5]
  Demux/5 -> [phi_beta_hat_v5]
  S-Function/1 -> Demux/1
  [b_alpha_v5] -> Mux10/4
  Demux/2 -> [beta_hat_v5]
  [beta_noise_v5] -> Mux10/2
  [miu_noise_v5] -> Mux10/3
  [b_beta_v5] -> Mux10/5

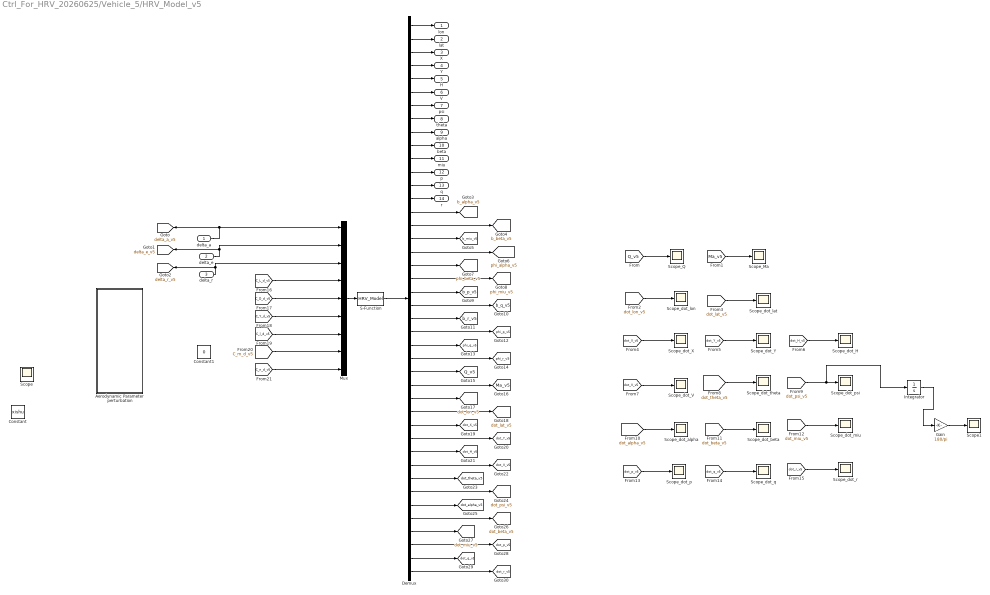
== system Ctrl_For_HRV_20260625/Vehicle_5/HRV_Model_v5 ==
  delta_a : Inport
  delta_e : Inport  Port=2
  delta_r : Inport  Port=3
  Aerodynamic Parameter perturbation : Subsystem
  Constant : Constant  Value=xishu  SampleTime=-1
  Constant1 : Constant  Value=0
  Demux : Demux  Outputs=14 + 12 + 2 + 14
  Gain : Gain  Gain=180/pi
  Integrator : Integrator  InitialCondition=[0 0 900 700 0 0 0.0698131700797732 0 0 0 0 0 0 0 0 0 0 0 0 0 0 0 0 0 0 0 0 0 0 0 0 0 0 0 0 0 0 0 0 0 0 0]
  Mux : Mux  Inputs=9
  S-Function : S-Function  FunctionName=HRV_Model  SFunctionDeploymentMode=off  EnableBusSupport=off
  Scope : Scope
  Scope1 : Scope
  Scope_Ma : Scope
  Scope_Q : Scope
  Scope_dot_H : Scope
  Scope_dot_V : Scope
  Scope_dot_X : Scope
  Scope_dot_Y : Scope
  Scope_dot_alpha : Scope
  Scope_dot_beta : Scope
  Scope_dot_lat : Scope
  Scope_dot_lon : Scope
  Scope_dot_miu : Scope
  Scope_dot_p : Scope
  Scope_dot_psi : Scope
  Scope_dot_q : Scope
  Scope_dot_r : Scope
  Scope_dot_theta : Scope
  lon : Outport
  lat : Outport  Port=2
  X : Outport  Port=3
  Y : Outport  Port=4
  H : Outport  Port=5
  V : Outport  Port=6
  psi : Outport  Port=7
  theta : Outport  Port=8
  alpha : Outport  Port=9
  beta : Outport  Port=10
  miu : Outport  Port=11
  p : Outport  Port=12
  q : Outport  Port=13
  r : Outport  Port=14
  tag scope: Ma_v5=global, Q_v5=global, b_alpha_v5=global, b_beta_v5=global, b_miu_v5=global, b_p_v5=global, b_q_v5=global, b_r_v5=global, delta_a_v5=global, delta_e_v5=global, delta_r_v5=global, dot_H_v5=global, dot_V_v5=global, dot_X_v5=global, dot_Y_v5=global, dot_alpha_v5=global, dot_beta_v5=global, dot_lat_v5=global, dot_lon_v5=global, dot_miu_v5=global, dot_p_v5=global, dot_psi_v5=global, dot_q_v5=global, dot_r_v5=global, dot_theta_v5=global, phi_alpha_v5=global, phi_beta_v5=global, phi_miu_v5=global, phi_p_v5=global, phi_q_v5=global, phi_r_v5=global
  wires:
  Gain/1 -> Scope1/1
  Integrator/1 -> Gain/1
  [C_n_d_v5] -> Mux/9
  [C_m_d_v5] -> Mux/8
  [C_l_d_v5] -> Mux/7
  [C_Y_d_v5] -> Mux/6
  [C_D_d_v5] -> Mux/5
  [C_L_d_v5] -> Mux/4
  [dot_p_v5] -> Scope_dot_p/1
  [dot_q_v5] -> Scope_dot_q/1
  [dot_r_v5] -> Scope_dot_r/1
  [dot_miu_v5] -> Scope_dot_miu/1
  [dot_beta_v5] -> Scope_dot_beta/1
  [dot_alpha_v5] -> Scope_dot_alpha/1
  [dot_psi_v5] -> Scope_dot_psi/1, Integrator/1
  [dot_theta_v5] -> Scope_dot_theta/1
  [dot_V_v5] -> Scope_dot_V/1
  [dot_H_v5] -> Scope_dot_H/1
  [dot_Y_v5] -> Scope_dot_Y/1
  [dot_X_v5] -> Scope_dot_X/1
  [dot_lat_v5] -> Scope_dot_lat/1
  [dot_lon_v5] -> Scope_dot_lon/1
  [Ma_v5] -> Scope_Ma/1
  [Q_v5] -> Scope_Q/1
  Demux/42 -> [dot_r_v5]
  Demux/41 -> [dot_q_v5]
  Demux/40 -> [dot_p_v5]
  Demux/38 -> [dot_beta_v5]
  Demux/39 -> [dot_miu_v5]
  Demux/33 -> [dot_H_v5]
  Demux/35 -> [dot_theta_v5]
  Demux/34 -> [dot_V_v5]
  Demux/36 -> [dot_psi_v5]
  Demux/37 -> [dot_alpha_v5]
  Demux/32 -> [dot_Y_v5]
  Demux/31 -> [dot_X_v5]
  Demux/29 -> [dot_lon_v5]
  Demux/30 -> [dot_lat_v5]
  Demux/28 -> [Ma_v5]
  Demux/27 -> [Q_v5]
  Demux/26 -> [phi_r_v5]
  Demux/25 -> [phi_q_v5]
  Demux/24 -> [phi_p_v5]
  Demux/23 -> [b_r_v5]
  Demux/19 -> [phi_beta_v5]
  Demux/20 -> [phi_miu_v5]
  Demux/22 -> [b_q_v5]
  Demux/21 -> [b_p_v5]
  Demux/17 -> [b_miu_v5]
  Demux/18 -> [phi_alpha_v5]
  Demux/16 -> [b_beta_v5]
  Demux/15 -> [b_alpha_v5]
  Demux/4 -> Y/1
  delta_a/1 -> Mux/1, [delta_a_v5]
  Demux/13 -> q/1
  delta_r/1 -> Mux/3, [delta_r_v5]
  Demux/14 -> r/1
  Demux/6 -> V/1
  delta_e/1 -> Mux/2, [delta_e_v5]
  Demux/5 -> H/1
  Demux/12 -> p/1
  Demux/9 -> alpha/1
  Demux/10 -> beta/1
  Demux/11 -> miu/1
  Demux/7 -> psi/1
  Demux/3 -> X/1
  Demux/2 -> lat/1
  Demux/1 -> lon/1
  S-Function/1 -> Demux/1
  Mux/1 -> S-Function/1
  Demux/8 -> theta/1

== system Ctrl_For_HRV_20260625/Vehicle_5/PNG ==
  Delay : Delay  DelayLength=1
  Demux : Demux  Outputs=3
  MATLAB Function : MATLAB Function  TreatAsAtomicUnit=on
  MATLAB Function1 : MATLAB Function  TreatAsAtomicUnit=on  SystemSampleTime=0.02
  MATLAB Function2 : MATLAB Function  TreatAsAtomicUnit=on
  Mux : Mux  Inputs=7+2
  PNG : MATLABFcn  MATLABFcn=PNG_2026_6_23(u)  OutputDimensions=3
  Scope{,1..4} (5 alike) : Scope
  Scope5 : Scope  NumInputPorts=2
  tag scope: alpha_cmd=global, f_psi=global, miu_cmd=global
  wires:
  Delay/1 -> MATLAB Function1/6(miu_last)
  [theta] -> Mux/9
  [f_psi] -> Mux/8
  MATLAB Function2/1(f_psi) -> [f_psi]
  [H] -> MATLAB Function2/5(H)
  [lat] -> MATLAB Function2/4(lat)
  [psi] -> MATLAB Function2/3(psi)
  [theta] -> MATLAB Function2/2(theta)
  [V] -> MATLAB Function2/1(V)
  Demux/3 -> Scope5/1
  [Q] -> Mux/7
  MATLAB Function1/2(miu_cmd) -> [miu_cmd], Scope3/1, Delay/1
  MATLAB Function1/1(alpha_cmd) -> [alpha_cmd], Scope2/1
  [Ma] -> MATLAB Function1/5(Ma)
  [H] -> MATLAB Function1/4(H)
  [Q] -> MATLAB Function1/3(Q)
  [nz_cmd] -> MATLAB Function1/2(nz_cmd)
  [ny_cmd] -> MATLAB Function1/1(ny_cmd)
  [nz_cmd] -> Scope1/1
  [ny_cmd] -> Scope/1
  Demux/2 -> [nz_cmd], Scope5/2
  Demux/1 -> [ny_cmd]
  PNG/1 -> Demux/1
  [V_target] -> Mux/6
  [Position_target] -> Mux/5
  MATLAB Function/1(v) -> Mux/4, Scope4/1
  [psi] -> MATLAB Function/3(psi)
  [theta] -> MATLAB Function/2(theta)
  [V] -> MATLAB Function/1(V)
  [H] -> Mux/3
  [Y] -> Mux/2
  [X] -> Mux/1
  Mux/1 -> PNG/1

== system Ctrl_For_HRV_20260625/Vehicle_5/actuator1_v5 ==
  delta_e_d : Inport
  Gain : Gain  Gain=50
  Integrator : Integrator
  Saturation : Saturate  UpperLimit=90  LowerLimit=-90
  Saturation1 : Saturate  UpperLimit=30  LowerLimit=-30
  Sum : Sum  Inputs=|+-
  delta_e : Outport
  wires:
  Saturation/1 -> Integrator/1
  Sum/1 -> Gain/1
  Integrator/1 -> Saturation1/1, Sum/2
  delta_e_d/1 -> Sum/1
  Gain/1 -> Saturation/1
  Saturation1/1 -> delta_e/1

== system Ctrl_For_HRV_20260625/Vehicle_5/actuator2_v5 ==
  delta_r_d : Inport
  Gain : Gain  Gain=50
  Integrator : Integrator
  Saturation : Saturate  UpperLimit=90  LowerLimit=-90
  Saturation1 : Saturate  UpperLimit=30  LowerLimit=-30
  Sum : Sum  Inputs=|+-
  delta_r : Outport
  wires:
  Saturation1/1 -> delta_r/1
  Gain/1 -> Saturation/1
  delta_r_d/1 -> Sum/1
  Integrator/1 -> Sum/2, Saturation1/1
  Sum/1 -> Gain/1
  Saturation/1 -> Integrator/1

== system Ctrl_For_HRV_20260625/Vehicle_5/actuator_v5 ==
  delta_a_d : Inport
  Gain : Gain  Gain=50
  Integrator : Integrator
  Saturation : Saturate  UpperLimit=90  LowerLimit=-90
  Saturation1 : Saturate  UpperLimit=30  LowerLimit=-30
  Sum : Sum  Inputs=|+-
  delta_a : Outport
  wires:
  Saturation1/1 -> delta_a/1
  Gain/1 -> Saturation/1
  delta_a_d/1 -> Sum/1
  Integrator/1 -> Sum/2, Saturation1/1
  Sum/1 -> Gain/1
  Saturation/1 -> Integrator/1

== system Ctrl_For_HRV_20260625/Vehicle_1/AngleRate_Controller_v1/TD_p ==
  note: z12
  note: z11
  p_d : Inport
  Add2 : Sum  Inputs=+-
  Constant : Constant  Value=r_p
  Constant1 : Constant  Value=h_p
  Integrator : Integrator
  Integrator1 : Integrator
  MATLAB Fcn1 : MATLABFcn  MATLABFcn=fhan(u(1),u(2),u(3),u(4))
  Mux : Mux
  p_c : Outport  VectorParamsAs1DForOutWhenUnconnected=off
  p_c_dot : Outport  Port=2  VectorParamsAs1DForOutWhenUnconnected=off
  wires:
  p_d/1 -> Add2/2
  Add2/1 -> Mux/1
  Constant1/1 -> Mux/4
  Constant/1 -> Mux/3
  Mux/1 -> MATLAB Fcn1/1
  MATLAB Fcn1/1 -> Integrator/1
  Integrator1/1 -> p_c/1, Add2/1
  Integrator/1 -> Mux/2, p_c_dot/1, Integrator1/1

== system Ctrl_For_HRV_20260625/Vehicle_1/AngleRate_Controller_v1/TD_q ==
  note: z12
  note: z11
  q_d : Inport
  Add2 : Sum  Inputs=+-
  Constant : Constant  Value=r_q
  Constant1 : Constant  Value=h_q
  Integrator : Integrator
  Integrator1 : Integrator
  MATLAB Fcn1 : MATLABFcn  MATLABFcn=fhan(u(1),u(2),u(3),u(4))
  Mux : Mux
  q_c : Outport  VectorParamsAs1DForOutWhenUnconnected=off
  q_c_dot : Outport  Port=2  VectorParamsAs1DForOutWhenUnconnected=off
  wires:
  q_d/1 -> Add2/2
  Add2/1 -> Mux/1
  Constant1/1 -> Mux/4
  Constant/1 -> Mux/3
  Mux/1 -> MATLAB Fcn1/1
  MATLAB Fcn1/1 -> Integrator/1
  Integrator1/1 -> q_c/1, Add2/1
  Integrator/1 -> Mux/2, q_c_dot/1, Integrator1/1

== system Ctrl_For_HRV_20260625/Vehicle_1/AngleRate_Controller_v1/TD_r ==
  note: z12
  note: z11
  r_d : Inport
  Add2 : Sum  Inputs=+-
  Constant : Constant  Value=r_r
  Constant1 : Constant  Value=h_r
  Integrator : Integrator
  Integrator1 : Integrator
  MATLAB Fcn1 : MATLABFcn  MATLABFcn=fhan(u(1),u(2),u(3),u(4))
  Mux : Mux
  r_c : Outport  VectorParamsAs1DForOutWhenUnconnected=off
  r_c_dot : Outport  Port=2  VectorParamsAs1DForOutWhenUnconnected=off
  wires:
  r_d/1 -> Add2/2
  Add2/1 -> Mux/1
  Constant1/1 -> Mux/4
  Constant/1 -> Mux/3
  Mux/1 -> MATLAB Fcn1/1
  MATLAB Fcn1/1 -> Integrator/1
  Integrator1/1 -> r_c/1, Add2/1
  Integrator/1 -> Mux/2, r_c_dot/1, Integrator1/1

== system Ctrl_For_HRV_20260625/Vehicle_1/Error_Model/TD_alpha1 ==
  note: z12
  note: z11
  e_wd_1 : Inport
  Add2 : Sum  Inputs=+-
  Constant : Constant  Value=r_alpha
  Constant1 : Constant  Value=h_alpha
  Integrator : Integrator
  Integrator1 : Integrator
  MATLAB Fcn1 : MATLABFcn  MATLABFcn=fhan(u(1),u(2),u(3),u(4))
  Mux : Mux
  dot_e_wd_1 : Outport  VectorParamsAs1DForOutWhenUnconnected=off
  wires:
  e_wd_1/1 -> Add2/2
  Add2/1 -> Mux/1
  Constant1/1 -> Mux/4
  Constant/1 -> Mux/3
  Mux/1 -> MATLAB Fcn1/1
  MATLAB Fcn1/1 -> Integrator/1
  Integrator1/1 -> Add2/1
  Integrator/1 -> Mux/2, dot_e_wd_1/1, Integrator1/1

== system Ctrl_For_HRV_20260625/Vehicle_1/Error_Model/TD_alpha2 ==
  note: z11
  note: z12
  e_wd_2 : Inport
  Add2 : Sum  Inputs=+-
  Constant : Constant  Value=r_alpha
  Constant1 : Constant  Value=h_alpha
  Integrator : Integrator
  Integrator1 : Integrator
  MATLAB Fcn1 : MATLABFcn  MATLABFcn=fhan(u(1),u(2),u(3),u(4))
  Mux : Mux
  dot_e_wd_2 : Outport  VectorParamsAs1DForOutWhenUnconnected=off
  wires:
  Integrator/1 -> Integrator1/1, dot_e_wd_2/1, Mux/2
  Integrator1/1 -> Add2/1
  MATLAB Fcn1/1 -> Integrator/1
  Mux/1 -> MATLAB Fcn1/1
  Constant/1 -> Mux/3
  Constant1/1 -> Mux/4
  Add2/1 -> Mux/1
  e_wd_2/1 -> Add2/2

== system Ctrl_For_HRV_20260625/Vehicle_1/Error_Model/TD_alpha3 ==
  note: z12
  note: z11
  e_wd_3 : Inport
  Add2 : Sum  Inputs=+-
  Constant : Constant  Value=r_alpha
  Constant1 : Constant  Value=h_alpha
  Integrator : Integrator
  Integrator1 : Integrator
  MATLAB Fcn1 : MATLABFcn  MATLABFcn=fhan(u(1),u(2),u(3),u(4))
  Mux : Mux
  dot_e_wd_3 : Outport  VectorParamsAs1DForOutWhenUnconnected=off
  wires:
  e_wd_3/1 -> Add2/2
  Add2/1 -> Mux/1
  Constant1/1 -> Mux/4
  Constant/1 -> Mux/3
  Mux/1 -> MATLAB Fcn1/1
  MATLAB Fcn1/1 -> Integrator/1
  Integrator1/1 -> Add2/1
  Integrator/1 -> Mux/2, dot_e_wd_3/1, Integrator1/1

== system Ctrl_For_HRV_20260625/Vehicle_1/FlowAngle_Controller_v1/TD_alpha ==
  note: z12
  note: z11
  alpha_d : Inport
  Add2 : Sum  Inputs=+-
  Constant : Constant  Value=r_alpha
  Constant1 : Constant  Value=h_alpha
  Integrator : Integrator
  Integrator1 : Integrator
  MATLAB Fcn1 : MATLABFcn  MATLABFcn=fhan(u(1),u(2),u(3),u(4))
  Mux : Mux
  Scope : Scope
  alpha_c : Outport  VectorParamsAs1DForOutWhenUnconnected=off
  alpha_c_dot : Outport  Port=2  VectorParamsAs1DForOutWhenUnconnected=off
  wires:
  alpha_d/1 -> Add2/2
  Add2/1 -> Mux/1
  Constant1/1 -> Mux/4
  Constant/1 -> Mux/3
  Mux/1 -> MATLAB Fcn1/1
  MATLAB Fcn1/1 -> Integrator/1
  Integrator1/1 -> alpha_c/1, Scope/1, Add2/1
  Integrator/1 -> Mux/2, alpha_c_dot/1, Integrator1/1

== system Ctrl_For_HRV_20260625/Vehicle_1/FlowAngle_Controller_v1/TD_alpha2 ==
  alpha_d : Inport
  Gain17 : Gain  Gain=1.2
  Integrator : Integrator
  Sum : Sum  Inputs=|+-
  alpha_c : Outport
  alpha_c_dot : Outport  Port=2
  wires:
  alpha_d/1 -> Sum/1
  Sum/1 -> Gain17/1
  Integrator/1 -> Sum/2, alpha_c/1
  Gain17/1 -> Integrator/1, alpha_c_dot/1

== system Ctrl_For_HRV_20260625/Vehicle_1/FlowAngle_Controller_v1/TD_alpha3 ==
  note: z12
  note: z11
  dot_beta_c : Inport
  Add2 : Sum  Inputs=+-
  Constant : Constant  Value=r_alpha
  Constant1 : Constant  Value=h_alpha
  Integrator : Integrator
  Integrator1 : Integrator
  MATLAB Fcn1 : MATLABFcn  MATLABFcn=fhan(u(1),u(2),u(3),u(4))
  Mux : Mux
  ddot_beta_c : Outport  VectorParamsAs1DForOutWhenUnconnected=off
  wires:
  dot_beta_c/1 -> Add2/2
  Add2/1 -> Mux/1
  Constant1/1 -> Mux/4
  Constant/1 -> Mux/3
  Mux/1 -> MATLAB Fcn1/1
  MATLAB Fcn1/1 -> Integrator/1
  Integrator1/1 -> Add2/1
  Integrator/1 -> Mux/2, ddot_beta_c/1, Integrator1/1

== system Ctrl_For_HRV_20260625/Vehicle_1/FlowAngle_Controller_v1/TD_alpha4 ==
  note: z12
  note: z11
  dot_miu_c : Inport
  Add2 : Sum  Inputs=+-
  Constant : Constant  Value=r_alpha
  Constant1 : Constant  Value=h_alpha
  Integrator : Integrator
  Integrator1 : Integrator
  MATLAB Fcn1 : MATLABFcn  MATLABFcn=fhan(u(1),u(2),u(3),u(4))
  Mux : Mux
  ddot_miu_c : Outport  VectorParamsAs1DForOutWhenUnconnected=off
  wires:
  dot_miu_c/1 -> Add2/2
  Add2/1 -> Mux/1
  Constant1/1 -> Mux/4
  Constant/1 -> Mux/3
  Mux/1 -> MATLAB Fcn1/1
  MATLAB Fcn1/1 -> Integrator/1
  Integrator1/1 -> Add2/1
  Integrator/1 -> Mux/2, ddot_miu_c/1, Integrator1/1

== system Ctrl_For_HRV_20260625/Vehicle_1/FlowAngle_Controller_v1/TD_beta ==
  note: z12
  note: z11
  beta_d : Inport
  Add2 : Sum  Inputs=+-
  Constant : Constant  Value=r_beta
  Constant1 : Constant  Value=h_beta
  Integrator : Integrator
  Integrator1 : Integrator
  MATLAB Fcn1 : MATLABFcn  MATLABFcn=fhan(u(1),u(2),u(3),u(4))
  Mux : Mux
  beta_c : Outport  VectorParamsAs1DForOutWhenUnconnected=off
  beta_c_dot : Outport  Port=2  VectorParamsAs1DForOutWhenUnconnected=off
  wires:
  beta_d/1 -> Add2/2
  Add2/1 -> Mux/1
  Constant1/1 -> Mux/4
  Constant/1 -> Mux/3
  Mux/1 -> MATLAB Fcn1/1
  MATLAB Fcn1/1 -> Integrator/1
  Integrator1/1 -> beta_c/1, Add2/1
  Integrator/1 -> Mux/2, beta_c_dot/1, Integrator1/1

== system Ctrl_For_HRV_20260625/Vehicle_1/FlowAngle_Controller_v1/TD_beta1 ==
  miu_d : Inport
  Gain17 : Gain  Gain=0.8
  Integrator : Integrator
  Sum : Sum  Inputs=|+-
  miu_c : Outport
  miu_c_dot : Outport  Port=2
  wires:
  miu_d/1 -> Sum/1
  Sum/1 -> Gain17/1
  Integrator/1 -> Sum/2, miu_c/1
  Gain17/1 -> Integrator/1, miu_c_dot/1

== system Ctrl_For_HRV_20260625/Vehicle_1/FlowAngle_Controller_v1/TD_beta2 ==
  beta_d : Inport
  Gain17 : Gain  Gain=1.2
  Integrator : Integrator
  Sum : Sum  Inputs=|+-
  beta_c : Outport
  beta_c_dot : Outport  Port=2
  wires:
  Gain17/1 -> beta_c_dot/1, Integrator/1
  Integrator/1 -> beta_c/1, Sum/2
  Sum/1 -> Gain17/1
  beta_d/1 -> Sum/1

== system Ctrl_For_HRV_20260625/Vehicle_1/FlowAngle_Controller_v1/TD_dotalpha1 ==
  note: z12
  note: z11
  dot_alpha_c : Inport
  Add2 : Sum  Inputs=+-
  Constant : Constant  Value=r_alpha
  Constant1 : Constant  Value=h_alpha
  Integrator : Integrator
  Integrator1 : Integrator
  MATLAB Fcn1 : MATLABFcn  MATLABFcn=fhan(u(1),u(2),u(3),u(4))
  Mux : Mux
  ddot_alpha_c : Outport  VectorParamsAs1DForOutWhenUnconnected=off
  wires:
  dot_alpha_c/1 -> Add2/2
  Add2/1 -> Mux/1
  Constant1/1 -> Mux/4
  Constant/1 -> Mux/3
  Mux/1 -> MATLAB Fcn1/1
  MATLAB Fcn1/1 -> Integrator/1
  Integrator1/1 -> Add2/1
  Integrator/1 -> Mux/2, ddot_alpha_c/1, Integrator1/1

== system Ctrl_For_HRV_20260625/Vehicle_1/FlowAngle_Controller_v1/TD_miu ==
  note: z12
  note: z11
  miu_d : Inport
  Add2 : Sum  Inputs=+-
  Constant : Constant  Value=r_miu
  Constant1 : Constant  Value=h_miu
  Integrator : Integrator
  Integrator1 : Integrator
  MATLAB Fcn1 : MATLABFcn  MATLABFcn=fhan(u(1),u(2),u(3),u(4))
  Mux : Mux
  miu_c : Outport  VectorParamsAs1DForOutWhenUnconnected=off
  miu_c_dot : Outport  Port=2  VectorParamsAs1DForOutWhenUnconnected=off
  wires:
  miu_d/1 -> Add2/2
  Add2/1 -> Mux/1
  Constant1/1 -> Mux/4
  Constant/1 -> Mux/3
  Mux/1 -> MATLAB Fcn1/1
  MATLAB Fcn1/1 -> Integrator/1
  Integrator1/1 -> miu_c/1, Add2/1
  Integrator/1 -> Mux/2, miu_c_dot/1, Integrator1/1

== system Ctrl_For_HRV_20260625/Vehicle_1/HRV_Model_v1/Aerodynamic Parameter perturbation ==
  Band-Limited White Noise : simulink/Sources/Band-Limited White Noise  Cov=1e-6  Ts=2  seed=101
  Band-Limited White Noise1 : simulink/Sources/Band-Limited White Noise  Cov=1e-6  Ts=2  seed=102
  Band-Limited White Noise10 : simulink/Sources/Band-Limited White Noise  Cov=1e-10  Ts=2  seed=103
  Band-Limited White Noise11 : simulink/Sources/Band-Limited White Noise  Cov=1e-10  Ts=2  seed=104
  Band-Limited White Noise12 : simulink/Sources/Band-Limited White Noise  Cov=1e-10  Ts=2  seed=105
  Band-Limited White Noise13 : simulink/Sources/Band-Limited White Noise  Cov=1e-10  Ts=2  seed=106
  Band-Limited White Noise4 : simulink/Sources/Band-Limited White Noise  Cov=1e-6  Ts=2  seed=107
  Band-Limited White Noise5 : simulink/Sources/Band-Limited White Noise  Cov=1e-6  Ts=2  seed=108
  Band-Limited White Noise6 : simulink/Sources/Band-Limited White Noise  Cov=1e-6  Ts=2  seed=109
  Band-Limited White Noise7 : simulink/Sources/Band-Limited White Noise  Cov=1e-6  Ts=2  seed=110
  Band-Limited White Noise8 : simulink/Sources/Band-Limited White Noise  Cov=1e-10  Ts=2  seed=111
  Band-Limited White Noise9 : simulink/Sources/Band-Limited White Noise  Cov=1e-10  Ts=2  seed=112
  Demux : Demux  Outputs=12
  Integrator : Integrator  InitialCondition=[xishu_L_0,xishu_D_0,xishu_Y_0,xishu_l_0,xishu_m_0,xishu_n_0,0,0,0,0,0,0]
  MATLAB Function : MATLAB Function  TreatAsAtomicUnit=on
  Mux : Mux  Inputs=12
  Scope{1..6} (6 alike) : Scope
  To Workspace : ToWorkspace  VariableName=C_L_d_v1  SampleTime=-1
      settings: Save2DSignal=2-D array (concatenate along first dimension)
  To Workspace1 : ToWorkspace  VariableName=C_D_d_v1  SampleTime=-1
      settings: Save2DSignal=2-D array (concatenate along first dimension)
  To Workspace2 : ToWorkspace  VariableName=C_Y_d_v1  SampleTime=-1
      settings: Save2DSignal=2-D array (concatenate along first dimension)
  To Workspace3 : ToWorkspace  VariableName=C_l_d_v1  SampleTime=-1
      settings: Save2DSignal=2-D array (concatenate along first dimension)
  To Workspace4 : ToWorkspace  VariableName=C_m_d_v1  SampleTime=-1
      settings: Save2DSignal=2-D array (concatenate along first dimension)
  To Workspace5 : ToWorkspace  VariableName=C_n_d_v1  SampleTime=-1
      settings: Save2DSignal=2-D array (concatenate along first dimension)
  tag scope: C_D_d_v1=global, C_L_d_v1=global, C_Y_d_v1=global, C_l_d_v1=global, C_m_d_v1=global, C_n_d_v1=global
  wires:
  [C_n_d_v1] -> To Workspace5/1
  [C_m_d_v1] -> To Workspace4/1
  [C_l_d_v1] -> To Workspace3/1
  [C_Y_d_v1] -> To Workspace2/1
  [C_L_d_v1] -> To Workspace/1
  [C_D_d_v1] -> To Workspace1/1
  [C_D_d_v1] -> Scope1/1
  [C_L_d_v1] -> Scope6/1
  [C_l_d_v1] -> Scope3/1
  [C_n_d_v1] -> Scope5/1
  [C_m_d_v1] -> Scope4/1
  [C_Y_d_v1] -> Scope2/1
  Demux/6 -> [C_n_d_v1]
  Demux/5 -> [C_m_d_v1]
  Demux/4 -> [C_l_d_v1]
  Demux/3 -> [C_Y_d_v1]
  Demux/2 -> [C_D_d_v1]
  Demux/1 -> [C_L_d_v1]
  Integrator/1 -> MATLAB Function/1(state), Demux/1
  MATLAB Function/1(dot_state) -> Integrator/1
  Band-Limited White Noise13/1 -> Mux/12
  Band-Limited White Noise12/1 -> Mux/11
  Band-Limited White Noise11/1 -> Mux/10
  Band-Limited White Noise10/1 -> Mux/9
  Band-Limited White Noise9/1 -> Mux/8
  Band-Limited White Noise8/1 -> Mux/7
  Band-Limited White Noise7/1 -> Mux/6
  Band-Limited White Noise6/1 -> Mux/5
  Band-Limited White Noise4/1 -> Mux/3
  Band-Limited White Noise5/1 -> Mux/4
  Band-Limited White Noise1/1 -> Mux/2
  Band-Limited White Noise/1 -> Mux/1
  Mux/1 -> MATLAB Function/2(u)

== system Ctrl_For_HRV_20260625/Vehicle_2/AngleRate_Controller_v2/TD_p ==
  note: z12
  note: z11
  p_d : Inport
  Add2 : Sum  Inputs=+-
  Constant : Constant  Value=r_p
  Constant1 : Constant  Value=h_p
  Integrator : Integrator
  Integrator1 : Integrator
  MATLAB Fcn1 : MATLABFcn  MATLABFcn=fhan(u(1),u(2),u(3),u(4))
  Mux : Mux
  p_c : Outport  VectorParamsAs1DForOutWhenUnconnected=off
  p_c_dot : Outport  Port=2  VectorParamsAs1DForOutWhenUnconnected=off
  wires:
  p_d/1 -> Add2/2
  Add2/1 -> Mux/1
  Constant1/1 -> Mux/4
  Constant/1 -> Mux/3
  Mux/1 -> MATLAB Fcn1/1
  MATLAB Fcn1/1 -> Integrator/1
  Integrator1/1 -> p_c/1, Add2/1
  Integrator/1 -> Mux/2, p_c_dot/1, Integrator1/1

== system Ctrl_For_HRV_20260625/Vehicle_2/AngleRate_Controller_v2/TD_q ==
  note: z12
  note: z11
  q_d : Inport
  Add2 : Sum  Inputs=+-
  Constant : Constant  Value=r_q
  Constant1 : Constant  Value=h_q
  Integrator : Integrator
  Integrator1 : Integrator
  MATLAB Fcn1 : MATLABFcn  MATLABFcn=fhan(u(1),u(2),u(3),u(4))
  Mux : Mux
  q_c : Outport  VectorParamsAs1DForOutWhenUnconnected=off
  q_c_dot : Outport  Port=2  VectorParamsAs1DForOutWhenUnconnected=off
  wires:
  q_d/1 -> Add2/2
  Add2/1 -> Mux/1
  Constant1/1 -> Mux/4
  Constant/1 -> Mux/3
  Mux/1 -> MATLAB Fcn1/1
  MATLAB Fcn1/1 -> Integrator/1
  Integrator1/1 -> q_c/1, Add2/1
  Integrator/1 -> Mux/2, q_c_dot/1, Integrator1/1

== system Ctrl_For_HRV_20260625/Vehicle_2/AngleRate_Controller_v2/TD_r ==
  note: z12
  note: z11
  r_d : Inport
  Add2 : Sum  Inputs=+-
  Constant : Constant  Value=r_r
  Constant1 : Constant  Value=h_r
  Integrator : Integrator
  Integrator1 : Integrator
  MATLAB Fcn1 : MATLABFcn  MATLABFcn=fhan(u(1),u(2),u(3),u(4))
  Mux : Mux
  r_c : Outport  VectorParamsAs1DForOutWhenUnconnected=off
  r_c_dot : Outport  Port=2  VectorParamsAs1DForOutWhenUnconnected=off
  wires:
  r_d/1 -> Add2/2
  Add2/1 -> Mux/1
  Constant1/1 -> Mux/4
  Constant/1 -> Mux/3
  Mux/1 -> MATLAB Fcn1/1
  MATLAB Fcn1/1 -> Integrator/1
  Integrator1/1 -> r_c/1, Add2/1
  Integrator/1 -> Mux/2, r_c_dot/1, Integrator1/1

== system Ctrl_For_HRV_20260625/Vehicle_2/Error_Model/TD_alpha1 ==
  note: z12
  note: z11
  e_wd_1 : Inport
  Add2 : Sum  Inputs=+-
  Constant : Constant  Value=r_alpha
  Constant1 : Constant  Value=h_alpha
  Integrator : Integrator
  Integrator1 : Integrator
  MATLAB Fcn1 : MATLABFcn  MATLABFcn=fhan(u(1),u(2),u(3),u(4))
  Mux : Mux
  dot_e_wd_1 : Outport  VectorParamsAs1DForOutWhenUnconnected=off
  wires:
  e_wd_1/1 -> Add2/2
  Add2/1 -> Mux/1
  Constant1/1 -> Mux/4
  Constant/1 -> Mux/3
  Mux/1 -> MATLAB Fcn1/1
  MATLAB Fcn1/1 -> Integrator/1
  Integrator1/1 -> Add2/1
  Integrator/1 -> Mux/2, dot_e_wd_1/1, Integrator1/1

== system Ctrl_For_HRV_20260625/Vehicle_2/Error_Model/TD_alpha2 ==
  note: z11
  note: z12
  e_wd_2 : Inport
  Add2 : Sum  Inputs=+-
  Constant : Constant  Value=r_alpha
  Constant1 : Constant  Value=h_alpha
  Integrator : Integrator
  Integrator1 : Integrator
  MATLAB Fcn1 : MATLABFcn  MATLABFcn=fhan(u(1),u(2),u(3),u(4))
  Mux : Mux
  dot_e_wd_2 : Outport  VectorParamsAs1DForOutWhenUnconnected=off
  wires:
  Integrator/1 -> Integrator1/1, dot_e_wd_2/1, Mux/2
  Integrator1/1 -> Add2/1
  MATLAB Fcn1/1 -> Integrator/1
  Mux/1 -> MATLAB Fcn1/1
  Constant/1 -> Mux/3
  Constant1/1 -> Mux/4
  Add2/1 -> Mux/1
  e_wd_2/1 -> Add2/2
